simulink model "MB"  (R2018a)
settings: Solver=VariableStepAuto  StartTime=0.0  StopTime=50  RelTol=1e-3
InitFcn:
  | setParameters
libraries: simulink x1
settings Model: Creator=win10  LastModifiedBy=win10

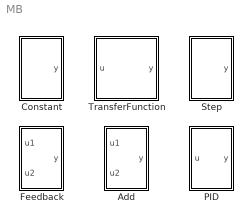
== system MB ==
  Add : Subsystem
  Constant : Subsystem  InitFcn=setParameters
  Feedback : Subsystem
  PID : Subsystem
  Step : Subsystem
  TransferFunction : Subsystem

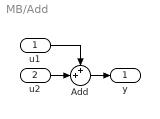
== system MB/Add ==
  u1 : Inport
  u2 : Inport  Port=2
  Add : Sum  Inputs=++|
  y : Outport
  wires:
  Add/1 -> y/1
  u1/1 -> Add/1
  u2/1 -> Add/2

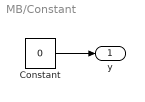
== system MB/Constant ==
  Constant : Constant  Value=0
  y : Outport
  wires:
  Constant/1 -> y/1

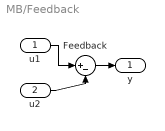
== system MB/Feedback ==
  u1 : Inport
  u2 : Inport  Port=2
  Feedback : Sum  Inputs=|+-
  y : Outport
  wires:
  u1/1 -> Feedback/1
  u2/1 -> Feedback/2
  Feedback/1 -> y/1

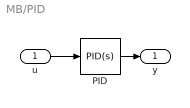
== system MB/PID ==
  u : Inport
  PID : simulink/Continuous/PID Controller  Controller=PID  TimeDomain=Continuous-time  SampleTime=-1  IntegratorMethod=Forward Euler  FilterMethod=Forward Euler  Form=Parallel  UseFilter=on  ControllerParametersSource=internal  P=1  I=1  D=0  N=1  InitialConditionSource=internal  InitialConditionForIntegrator=0  InitialConditionForFilter=0  ExternalReset=none  LimitOutput=off  UpperSaturationLimit=inf  LowerSaturationLimit=-inf  LinearizeAsGain=on  AntiWindupMode=none  Kb=1  TrackingMode=off  Kt=1  PParamMin=[]  PParamMax=[]  IParamMin=[]  IParamMax=[]  DParamMin=[]  DParamMax=[]  NParamMin=[]  NParamMax=[]  KbParamMin=[]  KbParamMax=[]  KtParamMin=[]  KtParamMax=[]  POutMin=[]  POutMax=[]  IOutMin=[]  IOutMax=[]  DOutMin=[]  DOutMax=[]  NOutMin=[]  NOutMax=[]  KbOutMin=[]  KbOutMax=[]  KtOutMin=[]  KtOutMax=[]  IntegratorOutMin=[]  IntegratorOutMax=[]  FilterOutMin=[]  FilterOutMax=[]  SumOutMin=[]  SumOutMax=[]  SumI1OutMin=[]  SumI1OutMax=[]  SumI2OutMin=[]  SumI2OutMax=[]  SumI3OutMin=[]  SumI3OutMax=[]  SumDOutMin=[]  SumDOutMax=[]  SaturationOutMin=[]  SaturationOutMax=[]  IntegratorContinuousStateAttributes=''  IntegratorStateMustResolveToSignalObject=off  IntegratorRTWStateStorageClass=Auto  FilterContinuousStateAttributes=''  FilterStateMustResolveToSignalObject=off  FilterRTWStateStorageClass=Auto  DifferentiatorICPrevScaledInput=0  DifferentiatorOutMin=[]  DifferentiatorOutMax=[]  FilterDiffOutCoefMin=[]  FilterDiffOutCoefMax=[]  SumDenOutMin=[]  SumDenOutMax=[]  SumNumOutMin=[]  SumNumOutMax=[]  ReciprocalOutMin=[]  ReciprocalOutMax=[]  DivideOutMin=[]  DivideOutMax=[]  TunerSelectOption=Transfer Function Based (PID Tuner App)
  y : Outport
  wires:
  PID/1 -> y/1
  u/1 -> PID/1

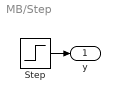
== system MB/Step ==
  Step : Step  Time=0.5  SampleTime=0
  y : Outport
  wires:
  Step/1 -> y/1

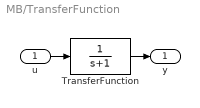
== system MB/TransferFunction ==
  u : Inport
  TransferFunction : TransferFcn  Denominator=[1 1]
  y : Outport
  wires:
  TransferFunction/1 -> y/1
  u/1 -> TransferFunction/1
